simulink model "sim_001"  (R2022a)
settings: Solver=VariableStepAuto  StartTime=0.0  StopTime=10  FixedStep=1e-5  MaxStep=1e-3  RelTol=1e-5
settings Model: Creator=Artun  LastModifiedBy=Artun
settings DebuggingCC: UnconnectedInputMsg=warning  UnconnectedOutputMsg=warning  UnconnectedLineMsg=warning
settings RTWCC: DLArmComputeVersion=19.05

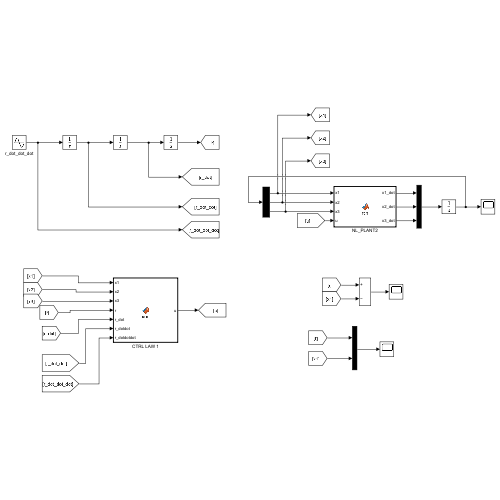
[thumbnail: Simulink's stored preview of the top-level diagram]
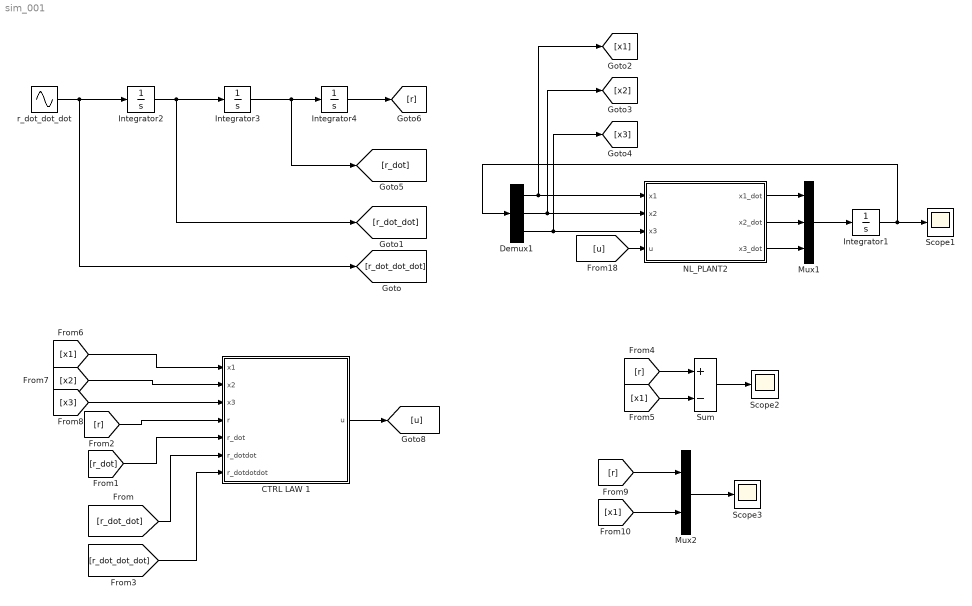
== system sim_001 ==
  CTRL LAW 1 : MATLAB Function  TreatAsAtomicUnit=on
  Demux1 : Demux  Outputs=3
  Integrator1 : Integrator  InitialCondition=ones(3,1)
  Integrator2 : Integrator
  Integrator3 : Integrator
  Integrator4 : Integrator
  Mux1 : Mux  Inputs=3
  Mux2 : Mux  Inputs=2
  NL_PLANT2 : MATLAB Function  TreatAsAtomicUnit=on
  Scope1 : Scope
  Scope2 : Scope
  Scope3 : Scope
  Sum : Sum  Inputs=+-
  r_dot_dot_dot : Sin  Frequency=2*pi*10  SampleTime=0
  wires:
  Integrator1/1 -> Demux1/1, Scope1/1
  Demux1/3 -> [x3], NL_PLANT2/3(x3)
  Demux1/2 -> [x2], NL_PLANT2/2(x2)
  Demux1/1 -> [x1], NL_PLANT2/1(x1)
  Mux1/1 -> Integrator1/1
  NL_PLANT2/3(x3_dot) -> Mux1/3
  NL_PLANT2/2(x2_dot) -> Mux1/2
  NL_PLANT2/1(x1_dot) -> Mux1/1
  [r] -> CTRL LAW 1/4(r)
  [r_dot] -> CTRL LAW 1/5(r_dot)
  CTRL LAW 1/1(u) -> [u]
  [u] -> NL_PLANT2/4(u)
  [r] -> Sum/1
  [x1] -> Sum/2
  Sum/1 -> Scope2/1
  r_dot_dot_dot/1 -> [r_dot_dot_dot], Integrator2/1
  Integrator2/1 -> [r_dot_dot], Integrator3/1
  Integrator3/1 -> [r_dot], Integrator4/1
  Integrator4/1 -> [r]
  [r_dot_dot] -> CTRL LAW 1/6(r_dotdot)
  [r_dot_dot_dot] -> CTRL LAW 1/7(r_dotdotdot)
  [x1] -> CTRL LAW 1/1(x1)
  [x2] -> CTRL LAW 1/2(x2)
  [x3] -> CTRL LAW 1/3(x3)
  [r] -> Mux2/1
  [x1] -> Mux2/2
  Mux2/1 -> Scope3/1

== matlab function sim_001/CTRL LAW 1 ==
  data: x1 input; x2 input; x3 input; r input; r_dot input; u output; r_dotdot input; r_dotdotdot input
function u = uuu(x1,x2,x3,r,r_dot,r_dotdot,r_dotdotdot)
u=3*r + 5*r_dot + 3*r_dotdot + r_dotdotdot ...
    - 3*x1 - 5*x2 - 3*x3- 6*x1*x2 - 2*x1*x3 ...
    - 5*x1^2 - 6*x1^3 - 2*x2^2 - 6*x1^4 - 8*x1^2*x2;
end

== matlab function sim_001/NL_PLANT2 ==
  data: x1 input; x2 input; x3 input; u input; x1_dot output; x2_dot output; x3_dot output
function [x1_dot, x2_dot, x3_dot] = fcn(x1, x2, x3, u)
x1_dot=(x1)^2+x2;
x2_dot=x3;
x3_dot=u;
end
